simulink model "racing_car_runge_dynamics"  (R2021b)
settings: Solver=VariableStepAuto  StartTime=0.0  StopTime=10.0  RelTol=1e-3
settings Model: Creator=KURAPAS  LastModifiedBy=KURAPAS

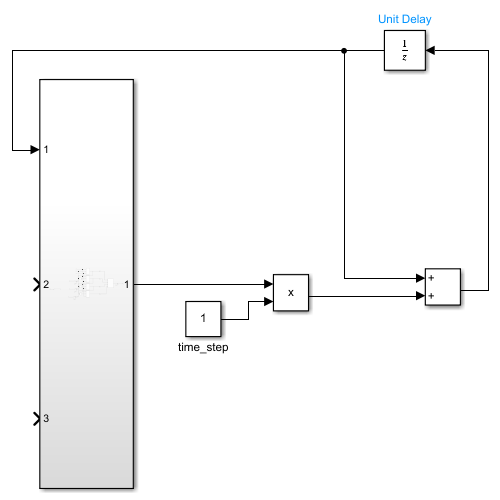
[thumbnail: Simulink's stored preview of the top-level diagram]
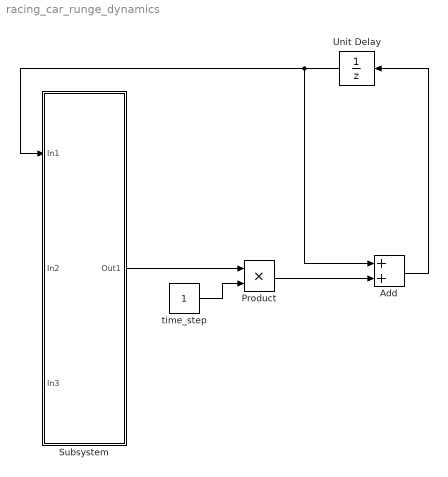
== system racing_car_runge_dynamics ==
  Add : Sum
  Product : Product
  Subsystem : Subsystem
  Unit Delay : UnitDelay  SampleTime=-1  HasFrameUpgradeWarning=on
  time_step : Constant
  wires:
  Subsystem/1(Out1) -> Product/1
  time_step/1 -> Product/2
  Product/1 -> Add/2
  Add/1 -> Unit Delay/1
  Unit Delay/1 -> Add/1, Subsystem/1(In1)

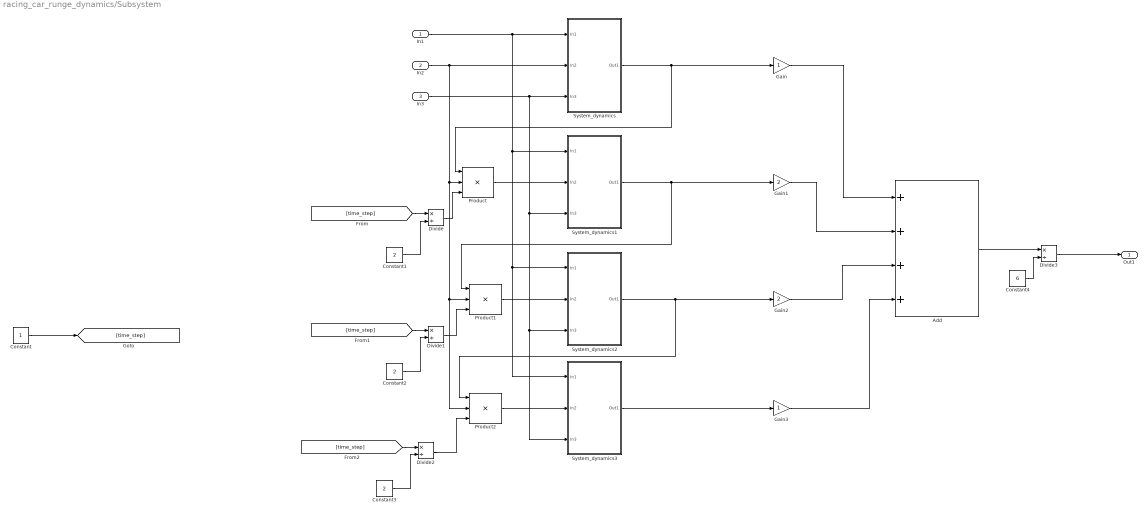
== system racing_car_runge_dynamics/Subsystem ==
  In1 : Inport
  In2 : Inport  Port=2
  In3 : Inport  Port=3
  Add : Sum  Inputs=++++
  Constant : Constant
  Constant1 : Constant  Value=2
  Constant2 : Constant  Value=2
  Constant3 : Constant  Value=2
  Constant4 : Constant  Value=6
  Divide{,1..3} (4 alike) : Product  Inputs=*/
  Gain : Gain
  Gain1 : Gain  Gain=2
  Gain2 : Gain  Gain=2
  Gain3 : Gain
  Product : Product  Inputs=3
  Product1 : Product  Inputs=3
  Product2 : Product  Inputs=3
  System_dynamics : Subsystem
  System_dynamics1 : Subsystem
  System_dynamics2 : Subsystem
  System_dynamics3 : Subsystem
  Out1 : Outport
  wires:
  System_dynamics/1(Out1) -> Product/1, Gain/1
  System_dynamics3/1(Out1) -> Gain3/1
  In1/1 -> System_dynamics1/1(In1), System_dynamics3/1(In1), System_dynamics2/1(In1), System_dynamics/1(In1)
  Constant/1 -> [time_step]
  [time_step] -> Divide/1
  Constant1/1 -> Divide/2
  Divide/1 -> Product/3
  Product/1 -> System_dynamics1/2(In2)
  Product1/1 -> System_dynamics2/2(In2)
  System_dynamics1/1(Out1) -> Gain1/1, Product1/1
  [time_step] -> Divide1/1
  Divide1/1 -> Product1/3
  Constant2/1 -> Divide1/2
  Divide2/1 -> Product2/3
  In2/1 -> System_dynamics/2(In2), Product/2, Product2/2, Product1/2
  Constant3/1 -> Divide2/2
  [time_step] -> Divide2/1
  System_dynamics2/1(Out1) -> Gain2/1, Product2/1
  Product2/1 -> System_dynamics3/2(In2)
  In3/1 -> System_dynamics3/3(In3), System_dynamics2/3(In3), System_dynamics1/3(In3), System_dynamics/3(In3)
  Gain/1 -> Add/1
  Gain1/1 -> Add/2
  Gain2/1 -> Add/3
  Gain3/1 -> Add/4
  Add/1 -> Divide3/1
  Constant4/1 -> Divide3/2
  Divide3/1 -> Out1/1

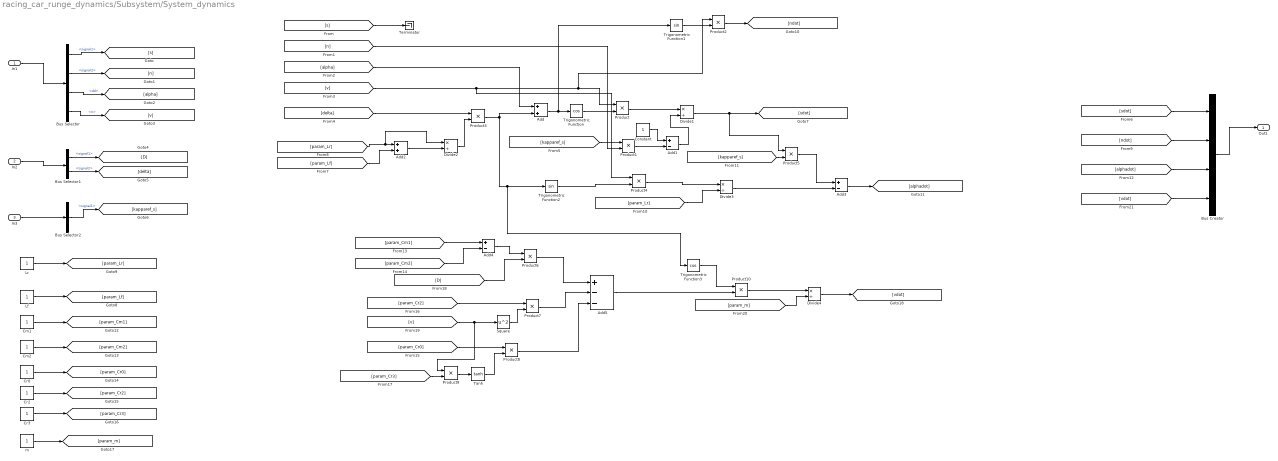
== system racing_car_runge_dynamics/Subsystem/System_dynamics ==
  In1 : Inport
  In2 : Inport  Port=2
  In3 : Inport  Port=3
  Add : Sum
  Add1 : Sum  Inputs=+-
  Add2 : Sum
  Add3 : Sum  Inputs=+-
  Add4 : Sum  Inputs=+-
  Add5 : Sum  Inputs=+--
  Bus Creator : BusCreator  Inputs=4
  Bus Selector : BusSelector  OutputSignals=signal1,signal2,dd,n
  Bus Selector1 : BusSelector  OutputSignals=signal1,signal2
  Bus Selector2 : BusSelector  OutputSignals=signal1
  Cm1 : Constant
  Cm2 : Constant
  Constant : Constant
  Cr0 : Constant
  Cr2 : Constant
  Cr3 : Constant
  Divide{1..4} (4 alike) : Product  Inputs=*/
  Lf : Constant
  Lr : Constant
  Product{,1..10} (11 alike) : Product
  Square : Math  Operator=square  SaturateOnIntegerOverflow=on
  Tanh : Trigonometry  Operator=tanh
  Terminator : Terminator
  Trigonometric Function : Trigonometry  Operator=cos
  Trigonometric Function1 : Trigonometry
  Trigonometric Function2 : Trigonometry
  Trigonometric Function3 : Trigonometry  Operator=cos
  m : Constant
  Out1 : Outport
  wires:
  In1/1 -> Bus Selector/1
  Bus Selector/1 -> [s]  "<signal1>"
  Bus Selector/2 -> [n]  "<signal2>"
  Bus Selector/3 -> [alpha]  "<dd>"
  Bus Selector/4 -> [v]  "<n>"
  Add/1 -> Trigonometric Function1/1, Trigonometric Function/1
  [alpha] -> Add/1
  In2/1 -> Bus Selector1/1
  Bus Selector1/1 -> [D]  "<signal1>"
  Bus Selector1/2 -> [delta]  "<signal2>"
  Trigonometric Function/1 -> Product/2
  [v] -> Product4/1, Product2/1, Product/1
  In3/1 -> Bus Selector2/1
  Bus Selector2/1 -> [kapparef_s]  "<signal1>"
  Constant/1 -> Add1/1
  [kapparef_s] -> Product1/1
  Product1/1 -> Add1/2
  [n] -> Product1/2
  Product/1 -> Divide1/1
  Add1/1 -> Divide1/2
  Divide1/1 -> Product5/1, [sdot]
  Bus Creator/1 -> Out1/1
  [sdot] -> Bus Creator/1
  Trigonometric Function1/1 -> Product2/2
  [param_Lr] -> Divide2/1, Add2/1
  [param_Lf] -> Add2/2
  Add2/1 -> Divide2/2
  [delta] -> Product3/1
  Divide2/1 -> Product3/2
  Lf/1 -> [param_Lf]
  Lr/1 -> [param_Lr]
  Product2/1 -> [ndot]
  [ndot] -> Bus Creator/2
  Trigonometric Function2/1 -> Product4/2
  Product4/1 -> Divide3/1
  [param_Lr] -> Divide3/2
  Product3/1 -> Add/2, Trigonometric Function3/1, Trigonometric Function2/1
  Divide3/1 -> Add3/2
  Product5/1 -> Add3/1
  [kapparef_s] -> Product5/2
  Add3/1 -> [alphadot]
  [alphadot] -> Bus Creator/3
  Cm1/1 -> [param_Cm1]
  Cm2/1 -> [param_Cm2]
  Cr0/1 -> [param_Cr0]
  Cr2/1 -> [param_Cr2]
  Cr3/1 -> [param_Cr3]
  [param_Cm1] -> Add4/1
  [param_Cm2] -> Add4/2
  Add4/1 -> Product6/1
  [D] -> Product6/2
  Product6/1 -> Add5/1
  [v] -> Product9/1, Square/1
  [param_Cr2] -> Product7/1
  Square/1 -> Product7/2
  Product7/1 -> Add5/2
  [param_Cr0] -> Product8/1
  Product9/1 -> Tanh/1
  Tanh/1 -> Product8/2
  Product8/1 -> Add5/3
  [param_Cr3] -> Product9/2
  [s] -> Terminator/1
  m/1 -> [param_m]
  Trigonometric Function3/1 -> Product10/1
  Add5/1 -> Product10/2
  Product10/1 -> Divide4/1
  [param_m] -> Divide4/2
  Divide4/1 -> [vdot]
  [vdot] -> Bus Creator/4

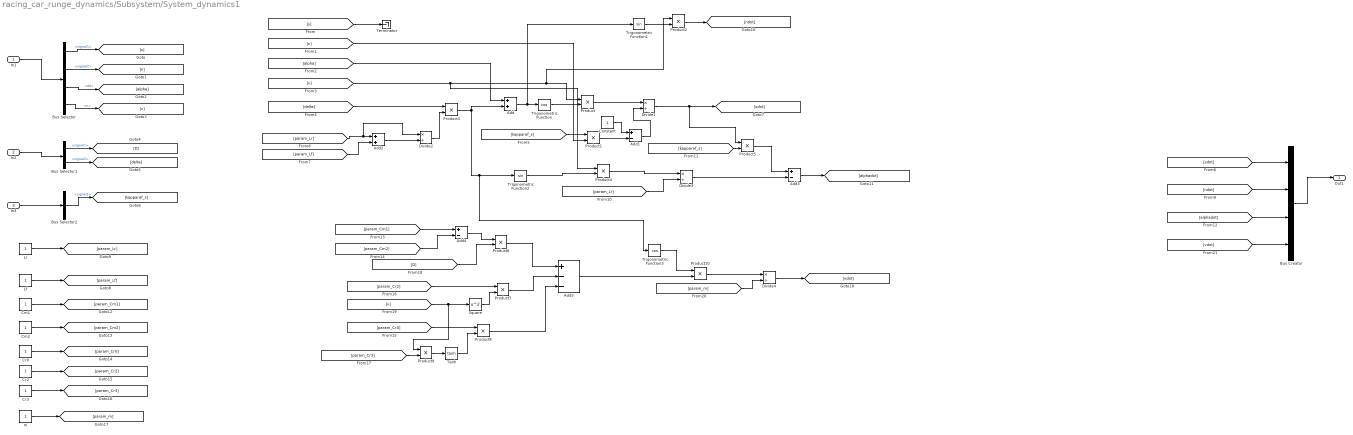
== system racing_car_runge_dynamics/Subsystem/System_dynamics1 ==
  In1 : Inport
  In2 : Inport  Port=2
  In3 : Inport  Port=3
  Add : Sum
  Add1 : Sum  Inputs=+-
  Add2 : Sum
  Add3 : Sum  Inputs=+-
  Add4 : Sum  Inputs=+-
  Add5 : Sum  Inputs=+--
  Bus Creator : BusCreator  Inputs=4
  Bus Selector : BusSelector  OutputSignals=signal1,signal2,dd,n
  Bus Selector1 : BusSelector  OutputSignals=signal1,signal2
  Bus Selector2 : BusSelector  OutputSignals=signal1
  Cm1 : Constant
  Cm2 : Constant
  Constant : Constant
  Cr0 : Constant
  Cr2 : Constant
  Cr3 : Constant
  Divide{1..4} (4 alike) : Product  Inputs=*/
  Lf : Constant
  Lr : Constant
  Product{,1..10} (11 alike) : Product
  Square : Math  Operator=square  SaturateOnIntegerOverflow=on
  Tanh : Trigonometry  Operator=tanh
  Terminator : Terminator
  Trigonometric Function : Trigonometry  Operator=cos
  Trigonometric Function1 : Trigonometry
  Trigonometric Function2 : Trigonometry
  Trigonometric Function3 : Trigonometry  Operator=cos
  m : Constant
  Out1 : Outport
  wires:
  In1/1 -> Bus Selector/1
  Bus Selector/1 -> [s]  "<signal1>"
  Bus Selector/2 -> [n]  "<signal2>"
  Bus Selector/3 -> [alpha]  "<dd>"
  Bus Selector/4 -> [v]  "<n>"
  Add/1 -> Trigonometric Function1/1, Trigonometric Function/1
  [alpha] -> Add/1
  In2/1 -> Bus Selector1/1
  Bus Selector1/1 -> [D]  "<signal1>"
  Bus Selector1/2 -> [delta]  "<signal2>"
  Trigonometric Function/1 -> Product/2
  [v] -> Product4/1, Product2/1, Product/1
  In3/1 -> Bus Selector2/1
  Bus Selector2/1 -> [kapparef_s]  "<signal1>"
  Constant/1 -> Add1/1
  [kapparef_s] -> Product1/1
  Product1/1 -> Add1/2
  [n] -> Product1/2
  Product/1 -> Divide1/1
  Add1/1 -> Divide1/2
  Divide1/1 -> Product5/1, [sdot]
  Bus Creator/1 -> Out1/1
  [sdot] -> Bus Creator/1
  Trigonometric Function1/1 -> Product2/2
  [param_Lr] -> Divide2/1, Add2/1
  [param_Lf] -> Add2/2
  Add2/1 -> Divide2/2
  [delta] -> Product3/1
  Divide2/1 -> Product3/2
  Lf/1 -> [param_Lf]
  Lr/1 -> [param_Lr]
  Product2/1 -> [ndot]
  [ndot] -> Bus Creator/2
  Trigonometric Function2/1 -> Product4/2
  Product4/1 -> Divide3/1
  [param_Lr] -> Divide3/2
  Product3/1 -> Add/2, Trigonometric Function3/1, Trigonometric Function2/1
  Divide3/1 -> Add3/2
  Product5/1 -> Add3/1
  [kapparef_s] -> Product5/2
  Add3/1 -> [alphadot]
  [alphadot] -> Bus Creator/3
  Cm1/1 -> [param_Cm1]
  Cm2/1 -> [param_Cm2]
  Cr0/1 -> [param_Cr0]
  Cr2/1 -> [param_Cr2]
  Cr3/1 -> [param_Cr3]
  [param_Cm1] -> Add4/1
  [param_Cm2] -> Add4/2
  Add4/1 -> Product6/1
  [D] -> Product6/2
  Product6/1 -> Add5/1
  [v] -> Product9/1, Square/1
  [param_Cr2] -> Product7/1
  Square/1 -> Product7/2
  Product7/1 -> Add5/2
  [param_Cr0] -> Product8/1
  Product9/1 -> Tanh/1
  Tanh/1 -> Product8/2
  Product8/1 -> Add5/3
  [param_Cr3] -> Product9/2
  [s] -> Terminator/1
  m/1 -> [param_m]
  Trigonometric Function3/1 -> Product10/1
  Add5/1 -> Product10/2
  Product10/1 -> Divide4/1
  [param_m] -> Divide4/2
  Divide4/1 -> [vdot]
  [vdot] -> Bus Creator/4

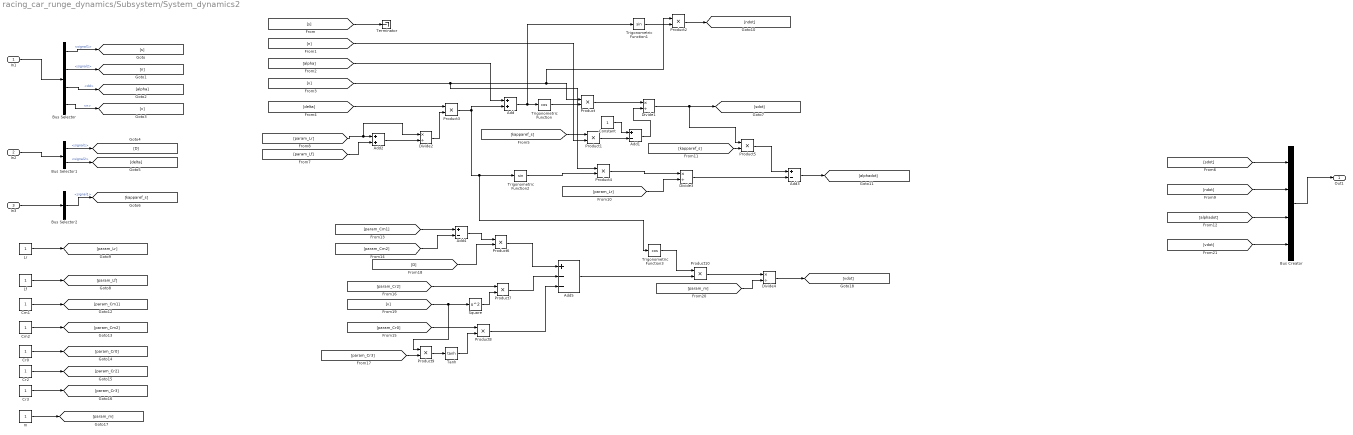
== system racing_car_runge_dynamics/Subsystem/System_dynamics2 ==
  In1 : Inport
  In2 : Inport  Port=2
  In3 : Inport  Port=3
  Add : Sum
  Add1 : Sum  Inputs=+-
  Add2 : Sum
  Add3 : Sum  Inputs=+-
  Add4 : Sum  Inputs=+-
  Add5 : Sum  Inputs=+--
  Bus Creator : BusCreator  Inputs=4
  Bus Selector : BusSelector  OutputSignals=signal1,signal2,dd,n
  Bus Selector1 : BusSelector  OutputSignals=signal1,signal2
  Bus Selector2 : BusSelector  OutputSignals=signal1
  Cm1 : Constant
  Cm2 : Constant
  Constant : Constant
  Cr0 : Constant
  Cr2 : Constant
  Cr3 : Constant
  Divide{1..4} (4 alike) : Product  Inputs=*/
  Lf : Constant
  Lr : Constant
  Product{,1..10} (11 alike) : Product
  Square : Math  Operator=square  SaturateOnIntegerOverflow=on
  Tanh : Trigonometry  Operator=tanh
  Terminator : Terminator
  Trigonometric Function : Trigonometry  Operator=cos
  Trigonometric Function1 : Trigonometry
  Trigonometric Function2 : Trigonometry
  Trigonometric Function3 : Trigonometry  Operator=cos
  m : Constant
  Out1 : Outport
  wires:
  In1/1 -> Bus Selector/1
  Bus Selector/1 -> [s]  "<signal1>"
  Bus Selector/2 -> [n]  "<signal2>"
  Bus Selector/3 -> [alpha]  "<dd>"
  Bus Selector/4 -> [v]  "<n>"
  Add/1 -> Trigonometric Function1/1, Trigonometric Function/1
  [alpha] -> Add/1
  In2/1 -> Bus Selector1/1
  Bus Selector1/1 -> [D]  "<signal1>"
  Bus Selector1/2 -> [delta]  "<signal2>"
  Trigonometric Function/1 -> Product/2
  [v] -> Product4/1, Product2/1, Product/1
  In3/1 -> Bus Selector2/1
  Bus Selector2/1 -> [kapparef_s]  "<signal1>"
  Constant/1 -> Add1/1
  [kapparef_s] -> Product1/1
  Product1/1 -> Add1/2
  [n] -> Product1/2
  Product/1 -> Divide1/1
  Add1/1 -> Divide1/2
  Divide1/1 -> Product5/1, [sdot]
  Bus Creator/1 -> Out1/1
  [sdot] -> Bus Creator/1
  Trigonometric Function1/1 -> Product2/2
  [param_Lr] -> Divide2/1, Add2/1
  [param_Lf] -> Add2/2
  Add2/1 -> Divide2/2
  [delta] -> Product3/1
  Divide2/1 -> Product3/2
  Lf/1 -> [param_Lf]
  Lr/1 -> [param_Lr]
  Product2/1 -> [ndot]
  [ndot] -> Bus Creator/2
  Trigonometric Function2/1 -> Product4/2
  Product4/1 -> Divide3/1
  [param_Lr] -> Divide3/2
  Product3/1 -> Add/2, Trigonometric Function3/1, Trigonometric Function2/1
  Divide3/1 -> Add3/2
  Product5/1 -> Add3/1
  [kapparef_s] -> Product5/2
  Add3/1 -> [alphadot]
  [alphadot] -> Bus Creator/3
  Cm1/1 -> [param_Cm1]
  Cm2/1 -> [param_Cm2]
  Cr0/1 -> [param_Cr0]
  Cr2/1 -> [param_Cr2]
  Cr3/1 -> [param_Cr3]
  [param_Cm1] -> Add4/1
  [param_Cm2] -> Add4/2
  Add4/1 -> Product6/1
  [D] -> Product6/2
  Product6/1 -> Add5/1
  [v] -> Product9/1, Square/1
  [param_Cr2] -> Product7/1
  Square/1 -> Product7/2
  Product7/1 -> Add5/2
  [param_Cr0] -> Product8/1
  Product9/1 -> Tanh/1
  Tanh/1 -> Product8/2
  Product8/1 -> Add5/3
  [param_Cr3] -> Product9/2
  [s] -> Terminator/1
  m/1 -> [param_m]
  Trigonometric Function3/1 -> Product10/1
  Add5/1 -> Product10/2
  Product10/1 -> Divide4/1
  [param_m] -> Divide4/2
  Divide4/1 -> [vdot]
  [vdot] -> Bus Creator/4

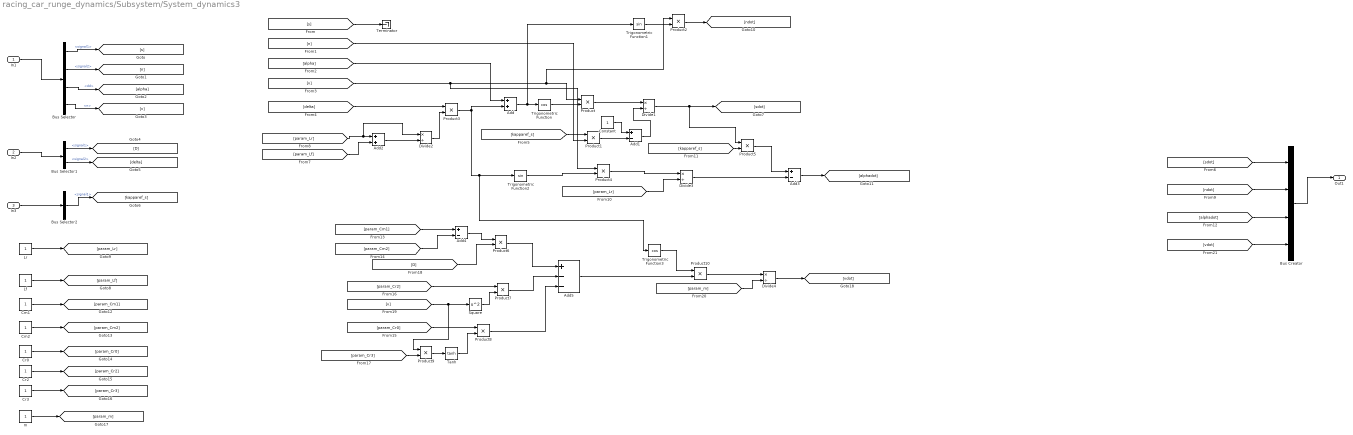
== system racing_car_runge_dynamics/Subsystem/System_dynamics3 ==
  In1 : Inport
  In2 : Inport  Port=2
  In3 : Inport  Port=3
  Add : Sum
  Add1 : Sum  Inputs=+-
  Add2 : Sum
  Add3 : Sum  Inputs=+-
  Add4 : Sum  Inputs=+-
  Add5 : Sum  Inputs=+--
  Bus Creator : BusCreator  Inputs=4
  Bus Selector : BusSelector  OutputSignals=signal1,signal2,dd,n
  Bus Selector1 : BusSelector  OutputSignals=signal1,signal2
  Bus Selector2 : BusSelector  OutputSignals=signal1
  Cm1 : Constant
  Cm2 : Constant
  Constant : Constant
  Cr0 : Constant
  Cr2 : Constant
  Cr3 : Constant
  Divide{1..4} (4 alike) : Product  Inputs=*/
  Lf : Constant
  Lr : Constant
  Product{,1..10} (11 alike) : Product
  Square : Math  Operator=square  SaturateOnIntegerOverflow=on
  Tanh : Trigonometry  Operator=tanh
  Terminator : Terminator
  Trigonometric Function : Trigonometry  Operator=cos
  Trigonometric Function1 : Trigonometry
  Trigonometric Function2 : Trigonometry
  Trigonometric Function3 : Trigonometry  Operator=cos
  m : Constant
  Out1 : Outport
  wires:
  In1/1 -> Bus Selector/1
  Bus Selector/1 -> [s]  "<signal1>"
  Bus Selector/2 -> [n]  "<signal2>"
  Bus Selector/3 -> [alpha]  "<dd>"
  Bus Selector/4 -> [v]  "<n>"
  Add/1 -> Trigonometric Function1/1, Trigonometric Function/1
  [alpha] -> Add/1
  In2/1 -> Bus Selector1/1
  Bus Selector1/1 -> [D]  "<signal1>"
  Bus Selector1/2 -> [delta]  "<signal2>"
  Trigonometric Function/1 -> Product/2
  [v] -> Product4/1, Product2/1, Product/1
  In3/1 -> Bus Selector2/1
  Bus Selector2/1 -> [kapparef_s]  "<signal1>"
  Constant/1 -> Add1/1
  [kapparef_s] -> Product1/1
  Product1/1 -> Add1/2
  [n] -> Product1/2
  Product/1 -> Divide1/1
  Add1/1 -> Divide1/2
  Divide1/1 -> Product5/1, [sdot]
  Bus Creator/1 -> Out1/1
  [sdot] -> Bus Creator/1
  Trigonometric Function1/1 -> Product2/2
  [param_Lr] -> Divide2/1, Add2/1
  [param_Lf] -> Add2/2
  Add2/1 -> Divide2/2
  [delta] -> Product3/1
  Divide2/1 -> Product3/2
  Lf/1 -> [param_Lf]
  Lr/1 -> [param_Lr]
  Product2/1 -> [ndot]
  [ndot] -> Bus Creator/2
  Trigonometric Function2/1 -> Product4/2
  Product4/1 -> Divide3/1
  [param_Lr] -> Divide3/2
  Product3/1 -> Add/2, Trigonometric Function3/1, Trigonometric Function2/1
  Divide3/1 -> Add3/2
  Product5/1 -> Add3/1
  [kapparef_s] -> Product5/2
  Add3/1 -> [alphadot]
  [alphadot] -> Bus Creator/3
  Cm1/1 -> [param_Cm1]
  Cm2/1 -> [param_Cm2]
  Cr0/1 -> [param_Cr0]
  Cr2/1 -> [param_Cr2]
  Cr3/1 -> [param_Cr3]
  [param_Cm1] -> Add4/1
  [param_Cm2] -> Add4/2
  Add4/1 -> Product6/1
  [D] -> Product6/2
  Product6/1 -> Add5/1
  [v] -> Product9/1, Square/1
  [param_Cr2] -> Product7/1
  Square/1 -> Product7/2
  Product7/1 -> Add5/2
  [param_Cr0] -> Product8/1
  Product9/1 -> Tanh/1
  Tanh/1 -> Product8/2
  Product8/1 -> Add5/3
  [param_Cr3] -> Product9/2
  [s] -> Terminator/1
  m/1 -> [param_m]
  Trigonometric Function3/1 -> Product10/1
  Add5/1 -> Product10/2
  Product10/1 -> Divide4/1
  [param_m] -> Divide4/2
  Divide4/1 -> [vdot]
  [vdot] -> Bus Creator/4
